simulink model "controlDahlin"  (R2023b)
settings: Solver=VariableStepAuto  StartTime=0.0  StopTime=200  RelTol=1e-3
settings Model: Creator=L03525615  LastModifiedBy=paulverdugo
settings DebuggingCC: UnconnectedInputMsg=warning  UnconnectedOutputMsg=warning  UnconnectedLineMsg=warning
settings ModelReferenceCC: EnableRefExpFcnMdlSchedulingChecks=on
settings RTWCC: DLArmComputeVersion=19.05

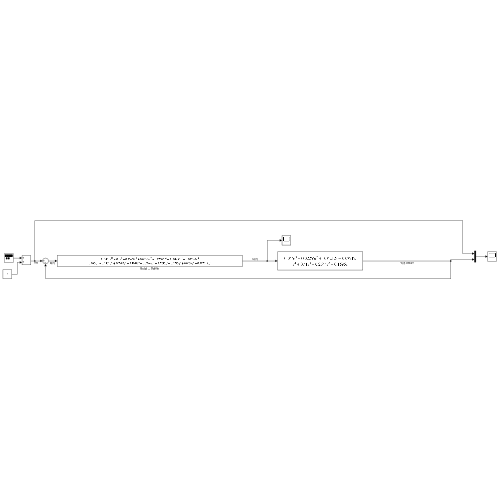
[thumbnail: Simulink's stored preview of the top-level diagram]
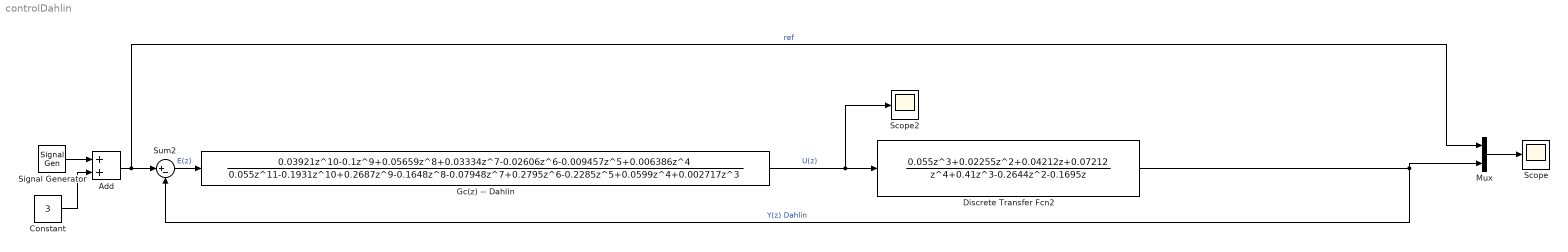
== system controlDahlin ==
  Add : Sum
  Constant : Constant  Value=3
  Discrete Transfer Fcn2 : DiscreteTransferFcn  Numerator=[0.055 0.02255 0.04212 0.07212]  Denominator=[1 0.41 -0.2644 -0.1695 0 ]  SampleTime=1
  "Gc(z) -- Dahlin" : DiscreteTransferFcn  Numerator=[0.03921 -0.1 0.05659 0.03334 -0.02606 -0.009457 0.006386 0 0 0 0]  Denominator=[0.055 -0.1931 0.2687 -0.1648 -0.07948 0.2795 -0.2285 0.0599 0.002717 0 0 0]  SampleTime=1
  Mux : Mux  Inputs=2
  Scope : Scope
  Scope2 : Scope
  Signal Generator : SignalGenerator  WaveForm=square  Amplitude=3  Frequency=0.2
  Sum2 : Sum  Inputs=|+-
  wires:
  Sum2/1 -> "Gc(z) -- Dahlin"/1  "E(z)"
  "Gc(z) -- Dahlin"/1 -> Scope2/1, Discrete Transfer Fcn2/1  "U(z)"
  Discrete Transfer Fcn2/1 -> Mux/2, Sum2/2  "Y(z) Dahlin"
  Mux/1 -> Scope/1
  Constant/1 -> Add/2
  Signal Generator/1 -> Add/1
  Add/1 -> Mux/1, Sum2/1  "ref"
